simulink model "Control Systems"  (R2024a)
settings: Solver=VariableStepAuto  StartTime=0.0  StopTime=12  MaxStep=0.01  RelTol=1e-3
values from neighbouring files (symbols this model uses):
  Dist_param = [mu,L,v]    [Param_init.m]
libraries: cstblocks x3, simulink x1, mpclib x1
settings Model: Creator=Buvaanesh  LastModifiedBy=Buvaanesh
settings RTWCC: GPUComputeCapability=3.5

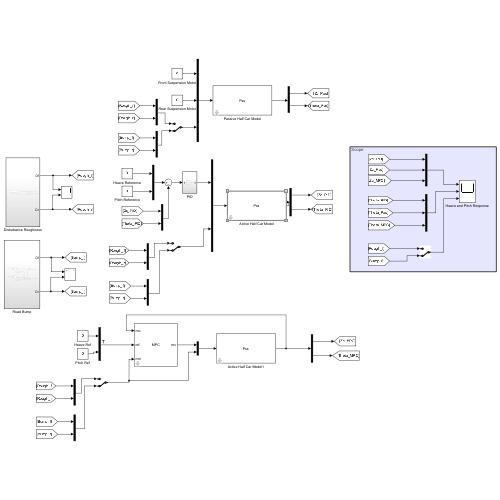
[thumbnail: Simulink's stored preview of the top-level diagram]
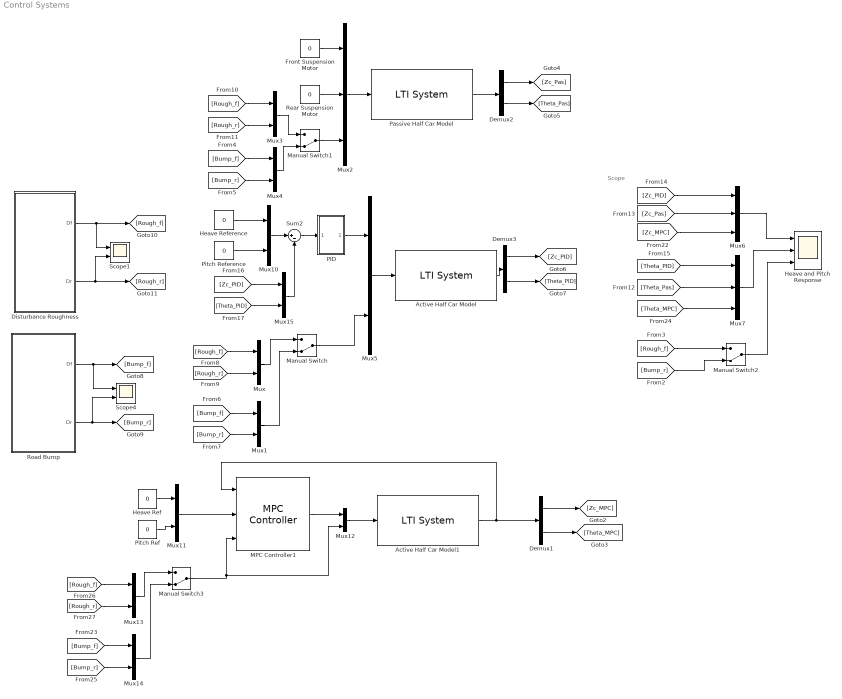
== system Control Systems ==
  note: Scope
  Active Half Car Model : cstblocks/LTI System  sys=Pss  IC=[0,0,0,0,0,0,0,0]  PadeOrder=0
  Active Half Car Model1 : cstblocks/LTI System  sys=Pss  IC=[0,0,0,0,0,0,0,0]  PadeOrder=0
  Demux1 : Demux  Outputs=2
  Demux2 : Demux  Outputs=2
  Demux3 : Demux  Outputs=2
  Disturbance Roughness : Subsystem
  Front Suspension Motor : Constant  Value=0
  Heave Ref : Constant  Value=0
  Heave Reference : Constant  Value=0
  Heave and Pitch Response : Scope  NumInputPorts=3
  MPC Controller1 : mpclib/MPC Controller  SCDEnableBlockLinearizationSpecification=on  mpcobj=mpc1  is_multiple=0  enable_value=0  return_u0=off  updateMPCinCallerWorkspace=on  md_inport=on  mv_inport=off  uref_inport=off  return_cost=off  return_mvseq=off  return_qpstatus=off  return_xseq=off  return_state=off  return_ovseq=off  state_inport=off  umin_inport=off  umax_inport=off  ymin_inport=off  ymax_inport=off  cc_inport=off  ywt_inport=off  uwt_inport=off  duwt_inport=off  rhoeps_inport=off  pm_inport=off  MaximumP=10  HorizonChoice=FixedHorizon  n_ts=0.01  n_p=100  n_mv=2  n_md=2  n_ud=0  n_mo=2  n_uo=0  BlockDataType=double  SampleTimeInherited=off  switch_inport=off
  Manual Switch{,1..3} (4 alike) : ManualSwitch  CurrentSetting=0
  Mux{,1,3..5,10..15} (11 alike) : Mux  Inputs=2
  Mux2 : Mux  Inputs=3
  Mux6 : Mux  Inputs=3
  Mux7 : Mux  Inputs=3
  PID : Subsystem
  Passive Half Car Model : cstblocks/LTI System  sys=Pss  IC=[0,0,0,0,0,0,0,0]  PadeOrder=0
  Pitch Ref : Constant  Value=0
  Pitch Reference : Constant  Value=0
  Rear Suspension Motor : Constant  Value=0
  Road Bump : Subsystem
  Scope1 : Scope  NumInputPorts=2
  Scope4 : Scope  NumInputPorts=2
  Sum2 : Sum  Inputs=|+-
  wires:
  Rear Suspension Motor/1 -> Mux2/2
  Front Suspension Motor/1 -> Mux2/1
  Passive Half Car Model/1 -> Demux2/1
  Mux2/1 -> Passive Half Car Model/1
  Pitch Reference/1 -> Mux10/2
  Active Half Car Model/1 -> Demux3/1
  Heave Reference/1 -> Mux10/1
  Demux2/1 -> [Zc_Pas]
  Demux2/2 -> [Theta_Pas]
  Demux3/1 -> [Zc_PID]
  Demux3/2 -> [Theta_PID]
  [Zc_PID] -> Mux15/1
  [Theta_PID] -> Mux15/2
  Mux7/1 -> Heave and Pitch Response/2
  [Theta_PID] -> Mux7/1
  [Zc_Pas] -> Mux6/2
  Mux6/1 -> Heave and Pitch Response/1
  [Theta_Pas] -> Mux7/2
  [Zc_PID] -> Mux6/1
  Road Bump/2(Dr) -> Scope4/2, [Bump_r]
  Road Bump/1(Df) -> Scope4/1, [Bump_f]
  Mux5/1 -> Active Half Car Model/1
  Disturbance Roughness/1(Df) -> Scope1/1, [Rough_f]
  Disturbance Roughness/2(Dr) -> [Rough_r], Scope1/2
  [Rough_f] -> Mux/1
  [Rough_r] -> Mux/2
  [Bump_f] -> Mux1/1
  [Bump_r] -> Mux1/2
  Mux/1 -> Manual Switch/1
  Mux1/1 -> Manual Switch/2
  Manual Switch/1 -> Mux5/2
  Mux4/1 -> Manual Switch1/2
  Mux3/1 -> Manual Switch1/1
  [Bump_r] -> Mux4/2
  [Bump_f] -> Mux4/1
  [Rough_r] -> Mux3/2
  [Rough_f] -> Mux3/1
  Manual Switch1/1 -> Mux2/3
  Manual Switch2/1 -> Heave and Pitch Response/3
  [Bump_r] -> Manual Switch2/2
  [Rough_f] -> Manual Switch2/1
  MPC Controller1/1 -> Mux12/1
  Heave Ref/1 -> Mux11/1
  Mux11/1 -> MPC Controller1/2
  Mux12/1 -> Active Half Car Model1/1
  Pitch Ref/1 -> Mux11/2
  Manual Switch3/1 -> MPC Controller1/3, Mux12/2
  Demux1/2 -> [Theta_MPC]
  Demux1/1 -> [Zc_MPC]
  Active Half Car Model1/1 -> MPC Controller1/1, Demux1/1
  [Zc_MPC] -> Mux6/3
  [Theta_MPC] -> Mux7/3
  Mux14/1 -> Manual Switch3/2
  Mux13/1 -> Manual Switch3/1
  [Bump_r] -> Mux14/2
  [Bump_f] -> Mux14/1
  [Rough_r] -> Mux13/2
  [Rough_f] -> Mux13/1
  Mux10/1 -> Sum2/1
  Mux15/1 -> Sum2/2
  PID/1(Out1) -> Mux5/1
  Sum2/1 -> PID/1(In1)

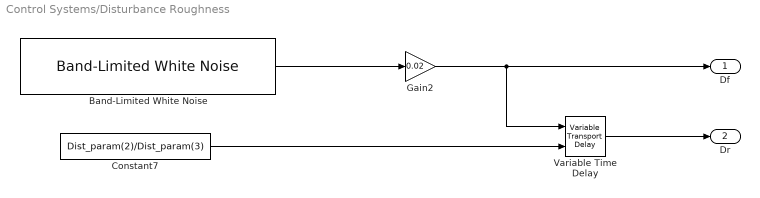
== system Control Systems/Disturbance Roughness ==
  Band-Limited White Noise : simulink/Sources/Band-Limited White Noise  Cov=[0.05]  Ts=0.05  seed=[23341]
  Constant7 : Constant  Value=Dist_param(2)/Dist_param(3)
  Gain2 : Gain  Gain=0.02
  Variable Time Delay : VariableTransportDelay  MaximumDelay=10  MaximumPoints=8182*100
  Df : Outport
  Dr : Outport  Port=2
  wires:
  Variable Time Delay/1 -> Dr/1
  Constant7/1 -> Variable Time Delay/2
  Band-Limited White Noise/1 -> Gain2/1
  Gain2/1 -> Variable Time Delay/1, Df/1

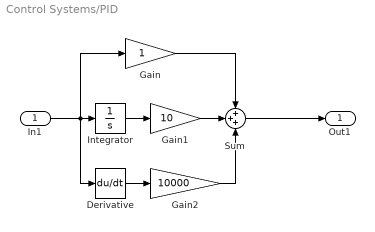
== system Control Systems/PID ==
  In1 : Inport
  Derivative : Derivative
  Gain : Gain
  Gain1 : Gain  Gain=10
  Gain2 : Gain  Gain=10000
  Integrator : Integrator
  Sum : Sum  Inputs=+++
  Out1 : Outport
  wires:
  In1/1 -> Derivative/1, Integrator/1, Gain/1
  Integrator/1 -> Gain1/1
  Gain/1 -> Sum/1
  Derivative/1 -> Gain2/1
  Sum/1 -> Out1/1
  Gain1/1 -> Sum/2
  Gain2/1 -> Sum/3

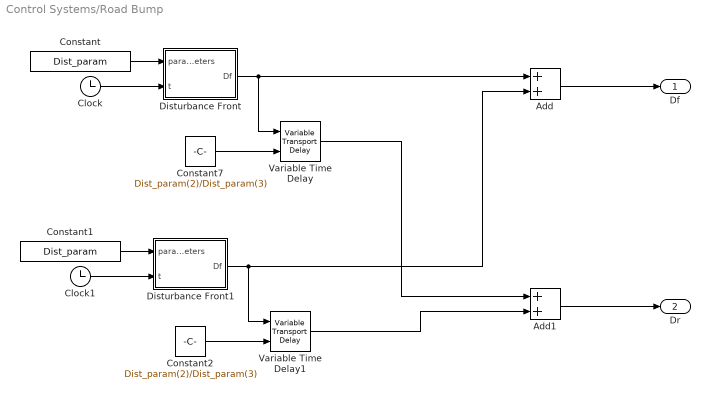
== system Control Systems/Road Bump ==
  Add : Sum
  Add1 : Sum
  Clock : Clock
      settings: Decimation=20
  Clock1 : Clock
      settings: Decimation=20
  Constant : Constant  Value=Dist_param
  Constant1 : Constant  Value=Dist_param
  Constant2 : Constant  Value=Dist_param(2)/Dist_param(3)
  Constant7 : Constant  Value=Dist_param(2)/Dist_param(3)
  Disturbance Front : MATLAB Function  TreatAsAtomicUnit=on
  Disturbance Front1 : MATLAB Function  TreatAsAtomicUnit=on
  Variable Time Delay : VariableTransportDelay  MaximumDelay=10  MaximumPoints=8192*100
  Variable Time Delay1 : VariableTransportDelay  MaximumDelay=10  MaximumPoints=8192*100
  Df : Outport
  Dr : Outport  Port=2
  wires:
  Constant7/1 -> Variable Time Delay/2
  Disturbance Front/1(Df) -> Variable Time Delay/1, Add/1
  Clock/1 -> Disturbance Front/2(t)
  Variable Time Delay/1 -> Add1/1
  Constant/1 -> Disturbance Front/1(parameters)
  Constant1/1 -> Disturbance Front1/1(parameters)
  Variable Time Delay1/1 -> Add1/2
  Clock1/1 -> Disturbance Front1/2(t)
  Disturbance Front1/1(Df) -> Add/2, Variable Time Delay1/1
  Constant2/1 -> Variable Time Delay1/2
  Add/1 -> Df/1
  Add1/1 -> Dr/1

== matlab function Control Systems/Road Bump/Disturbance Front1 ==
  data: parameters input; Df output; t input
function Df = fcn(parameters,t)

mu = parameters(1);

if (7.5<t) && (t<7.75)
    Df = -mu*(1-cos(8*pi*t));
else
    Df = 0;
end
end

== matlab function Control Systems/Road Bump/Disturbance Front ==
  data: parameters input; Df output; t input
function Df = fcn(parameters,t)

mu = parameters(1);

if (0.5<t) && (t<0.75)
    Df = mu*(1-cos(8*pi*t));
else
    Df = 0;
end
end
